simulink model "BMS_Software"  (R2025b)
settings: configuration reference "AutosarConfig" (kept outside this file)
undefined symbols (not defined in the file): BatteryNN, BMS_State_Enum, CntctWaitTime, Contact, currentFactor, CV_Gain, DiscIntNeverNeededParam, HighCellTempLimit, LowCellTempLimit, MaxCellVoltThrsld, MaxChrgCurrLimit, MaxDchrgCurrLimit, MinCellVoltDchrgCurrentLim_BP, MinCellVoltDchrgCurrentLim_Table, noCurrent, OverCellVoltageLimit, PlntBattNumCellPar, PlntBattNumCellSer, PreChrgTimeOut, PreChrgVoltRatio, SOCInit, SRE, ts, UnderCellVoltageLimit, voltThreshold
libraries: simulink x8, BatteryProtection x8, BatteryBalancing x1
settings Model: DataDictionary=BMS_Software_DD.sldd  EnableAccessToBaseWorkspace=off  PauseTimes=0  ExtModeTrigDuration=5  Creator=Chirag Patel  LastModifiedBy=smuckati
settings ConfigSetRef: SourceName=AutosarConfig

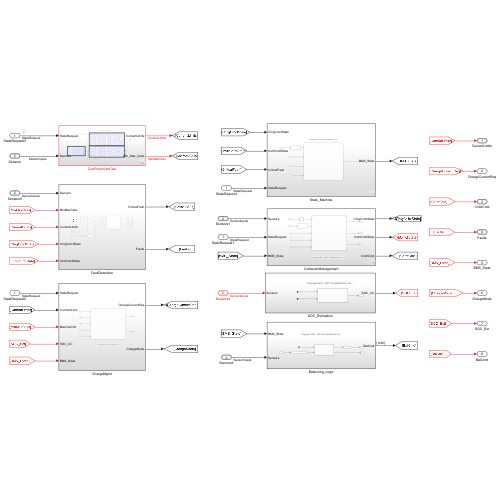
[thumbnail: Simulink's stored preview of the top-level diagram]
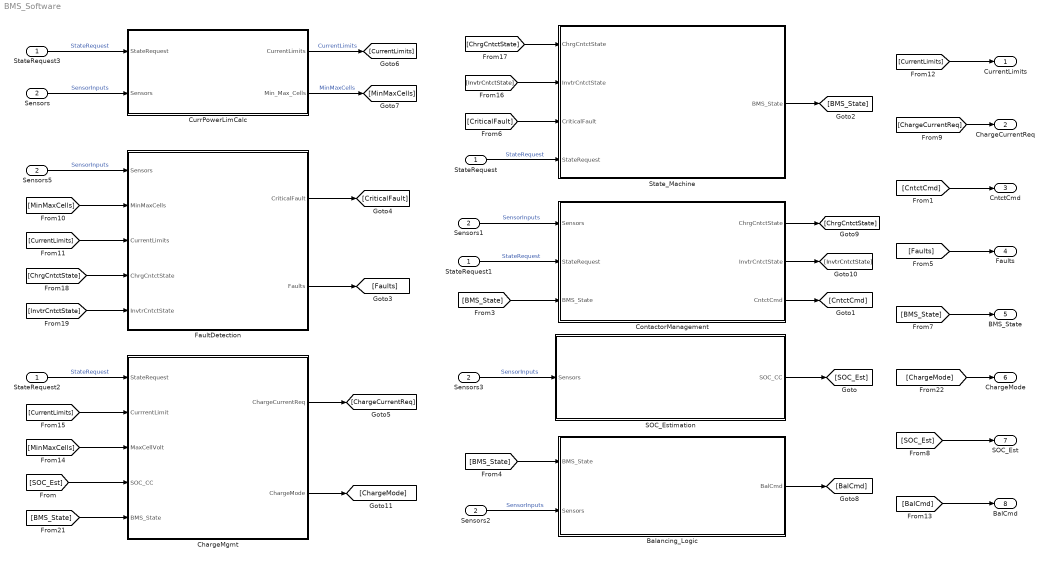
== system BMS_Software ==
  StateRequest : Inport  OutDataTypeStr=Enum: SRE  PortDimensions=1  SampleTime=ts
  Sensors : Inport  Port=2  OutDataTypeStr=Bus: Sensors  BusOutputAsStruct=on
  Balancing_Logic : Subsystem
  ChargeMgmt : Subsystem
  ContactorManagement : Subsystem
  CurrPowerLimCalc : Subsystem
  FaultDetection : Subsystem
  SOC_Estimation : Subsystem
  Sensors{1..3,5} (4 alike) : InportShadow  Port=2  OutDataTypeStr=Bus: Sensors  BusOutputAsStruct=on
  StateRequest1 : InportShadow  OutDataTypeStr=Enum: SRE  PortDimensions=1  SampleTime=ts
  StateRequest2 : InportShadow  OutDataTypeStr=Enum: SRE  PortDimensions=1  SampleTime=ts
  StateRequest3 : InportShadow  OutDataTypeStr=Enum: SRE  PortDimensions=1  SampleTime=ts
  State_Machine : Subsystem
  CurrentLimits : Outport  OutDataTypeStr=Bus: CurrentLimits
  ChargeCurrentReq : Outport  Port=2
  CntctCmd : Outport  Port=3  OutDataTypeStr=Bus: CntctCmd
  Faults : Outport  Port=4  OutDataTypeStr=Bus: Faults
  BMS_State : Outport  Port=5
  ChargeMode : Outport  Port=6
  SOC_Est : Outport  Port=7
  BalCmd : Outport  Port=8
  wires:
  Sensors3/1 -> SOC_Estimation/1(Sensors)  "SensorInputs"
  SOC_Estimation/1(SOC_CC) -> [SOC_Est]
  Sensors2/1 -> Balancing_Logic/2(Sensors)  "SensorInputs"
  [BMS_State] -> Balancing_Logic/1(BMS_State)
  StateRequest1/1 -> ContactorManagement/2(StateRequest)  "StateRequest"
  [BMS_State] -> ContactorManagement/3(BMS_State)
  [CntctCmd] -> CntctCmd/1
  Sensors/1 -> CurrPowerLimCalc/2(Sensors)  "SensorInputs"
  State_Machine/1(BMS_State) -> [BMS_State]
  [Faults] -> Faults/1
  ContactorManagement/3(CntctCmd) -> [CntctCmd]
  StateRequest/1 -> State_Machine/4(StateRequest)  "StateRequest"
  [BMS_State] -> BMS_State/1
  [ChargeCurrentReq] -> ChargeCurrentReq/1
  CurrPowerLimCalc/1(CurrentLimits) -> [CurrentLimits]  "CurrentLimits"
  CurrPowerLimCalc/2(Min_Max_Cells) -> [MinMaxCells]  "MinMaxCells"
  [CurrentLimits] -> CurrentLimits/1
  Balancing_Logic/1(BalCmd) -> [BalCmd]
  ContactorManagement/1(ChrgCntctState) -> [ChrgCntctState]
  ContactorManagement/2(InvtrCntctState) -> [InvtrCntctState]
  [MinMaxCells] -> ChargeMgmt/3(MaxCellVolt)
  [CurrentLimits] -> ChargeMgmt/2(CurrrentLimit)
  StateRequest2/1 -> ChargeMgmt/1(StateRequest)  "StateRequest"
  Sensors1/1 -> ContactorManagement/1(Sensors)  "SensorInputs"
  [SOC_Est] -> ChargeMgmt/4(SOC_CC)
  [ChrgCntctState] -> State_Machine/1(ChrgCntctState)
  [InvtrCntctState] -> State_Machine/2(InvtrCntctState)
  [CriticalFault] -> State_Machine/3(CriticalFault)
  ChargeMgmt/1(ChargeCurrentReq) -> [ChargeCurrentReq]
  ChargeMgmt/2(ChargeMode) -> [ChargeMode]
  [BMS_State] -> ChargeMgmt/5(BMS_State)
  [ChargeMode] -> ChargeMode/1
  [BalCmd] -> BalCmd/1
  [SOC_Est] -> SOC_Est/1
  FaultDetection/1(CriticalFault) -> [CriticalFault]
  FaultDetection/2(Faults) -> [Faults]
  [MinMaxCells] -> FaultDetection/2(MinMaxCells)
  Sensors5/1 -> FaultDetection/1(Sensors)  "SensorInputs"
  [CurrentLimits] -> FaultDetection/3(CurrentLimits)
  [ChrgCntctState] -> FaultDetection/4(ChrgCntctState)
  [InvtrCntctState] -> FaultDetection/5(InvtrCntctState)
  StateRequest3/1 -> CurrPowerLimCalc/1(StateRequest)  "StateRequest"

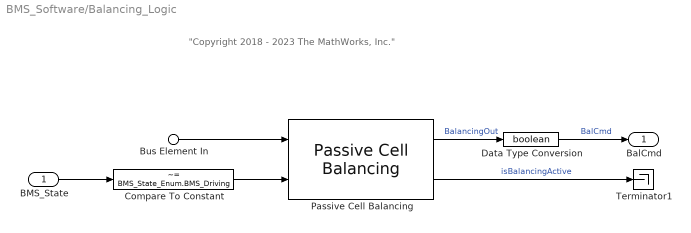
== system BMS_Software/Balancing_Logic ==
  note: "Copyright 2018 - 2023 The MathWorks, Inc."
  BMS_State : Inport  OutDataTypeStr=Enum: BMS_State_Enum  PortDimensions=1  SampleTime=[0.1,0]
  Bus Element In : Inport  Port=2  PortName=Sensors  Element=Cell_Voltages
  Compare To Constant : simulink/Logic and Bit Operations/Compare To Constant  relop=~=  const=BMS_State_Enum.BMS_Driving  OutDataTypeStr=boolean
  Data Type Conversion : DataTypeConversion  OutDataTypeStr=boolean  SaturateOnIntegerOverflow=off  RndMeth=Floor
  Passive Cell Balancing : BatteryBalancing/Passive Cell Balancing  Threshold=0.01  HysteresisBand=0  Td_on=20  Td_off=60  Ts=0.1  dataType=double
      settings: LibrarySourceBlock=batt_sl_lib/Cell Balancing/Passive Cell Balancing
  Terminator1 : Terminator
  BalCmd : Outport  OutDataTypeStr=boolean  PortDimensions=[1,PlntBattNumCellSer]  SampleTime=[0.1,0]  VectorParamsAs1DForOutWhenUnconnected=off
  wires:
  Data Type Conversion/1 -> BalCmd/1  "BalCmd"
  Compare To Constant/1 -> Passive Cell Balancing/2
  Bus Element In/1 -> Passive Cell Balancing/1
  Passive Cell Balancing/1 -> Data Type Conversion/1  "BalancingOut"
  Passive Cell Balancing/2 -> Terminator1/1  "isBalancingActive"
  BMS_State/1 -> Compare To Constant/1

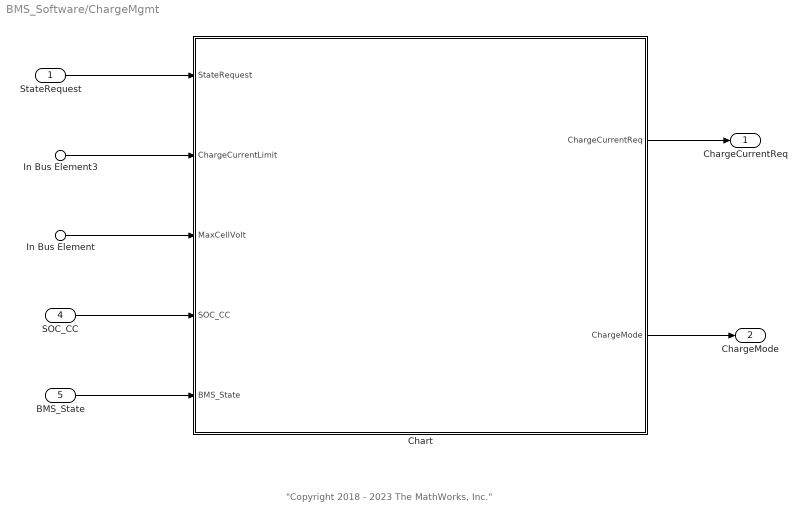
== system BMS_Software/ChargeMgmt ==
  note: "Copyright 2018 - 2023 The MathWorks, Inc."
  StateRequest : Inport  OutDataTypeStr=Enum: SRE  PortDimensions=1
  In Bus Element3 : Inport  Port=2  PortName=CurrrentLimit  Element=ChargeCurrentLimit
  In Bus Element : Inport  Port=3  PortName=MaxCellVolt  Element=MaxCellVolt
  SOC_CC : Inport  Port=4
  BMS_State : Inport  Port=5  OutDataTypeStr=Enum: BMS_State_Enum
  Chart : Stateflow chart  TreatAsAtomicUnit=on
  ChargeCurrentReq : Outport
  ChargeMode : Outport  Port=2
  wires:
  StateRequest/1 -> Chart/1(StateRequest)
  BMS_State/1 -> Chart/5(BMS_State)
  Chart/2(ChargeMode) -> ChargeMode/1
  In Bus Element/1 -> Chart/3(MaxCellVolt)
  Chart/1(ChargeCurrentReq) -> ChargeCurrentReq/1
  In Bus Element3/1 -> Chart/2(ChargeCurrentLimit)
  SOC_CC/1 -> Chart/4(SOC_CC)

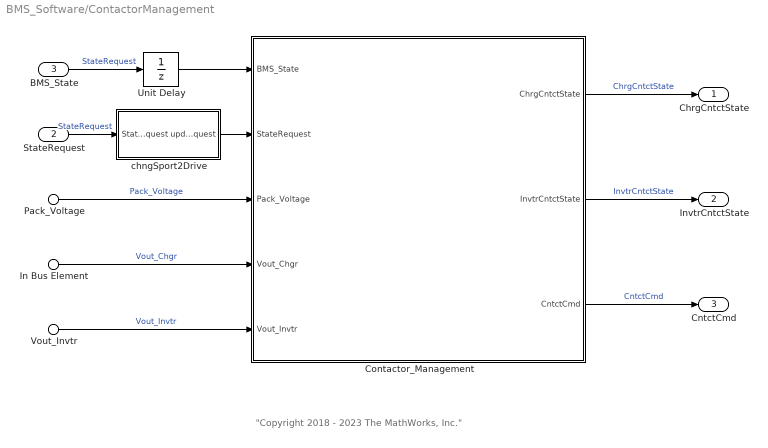
== system BMS_Software/ContactorManagement ==
  note: "Copyright 2018 - 2023 The MathWorks, Inc."
  Pack_Voltage : Inport  PortName=Sensors  Element=Pack_Voltage
  In Bus Element : Inport  PortName=Sensors  Element=Vout_Chgr
  Vout_Invtr : Inport  PortName=Sensors  Element=Vout_Invtr
  StateRequest : Inport  Port=2  OutDataTypeStr=Enum: SRE  PortDimensions=1  SampleTime=[0.10000000000000001,0]
  BMS_State : Inport  Port=3  OutDataTypeStr=Enum: BMS_State_Enum  PortDimensions=1  SampleTime=[0.10000000000000001,0]
  Contactor_Management : Stateflow chart  TreatAsAtomicUnit=on  VariantControl=(default)
  Unit Delay : UnitDelay  InitialCondition=BMS_State_Enum.BMS_Standby  SampleTime=-1  HasFrameUpgradeWarning=on
  chngSport2Drive : Subsystem
  ChrgCntctState : Outport
  InvtrCntctState : Outport  Port=2
  CntctCmd : Outport  Port=3  OutDataTypeStr=Bus: CntctCmd  BusOutputAsStruct=on
  wires:
  Unit Delay/1 -> Contactor_Management/1(BMS_State)
  Pack_Voltage/1 -> Contactor_Management/3(Pack_Voltage)  "Pack_Voltage"
  Vout_Invtr/1 -> Contactor_Management/5(Vout_Invtr)  "Vout_Invtr"
  Contactor_Management/3(CntctCmd) -> CntctCmd/1  "CntctCmd"
  Contactor_Management/1(ChrgCntctState) -> ChrgCntctState/1  "ChrgCntctState"
  In Bus Element/1 -> Contactor_Management/4(Vout_Chgr)  "Vout_Chgr"
  BMS_State/1 -> Unit Delay/1  "StateRequest"
  Contactor_Management/2(InvtrCntctState) -> InvtrCntctState/1  "InvtrCntctState"
  StateRequest/1 -> chngSport2Drive/1(StateRequest)  "StateRequest"
  chngSport2Drive/1(updatedStateRequest) -> Contactor_Management/2(StateRequest)

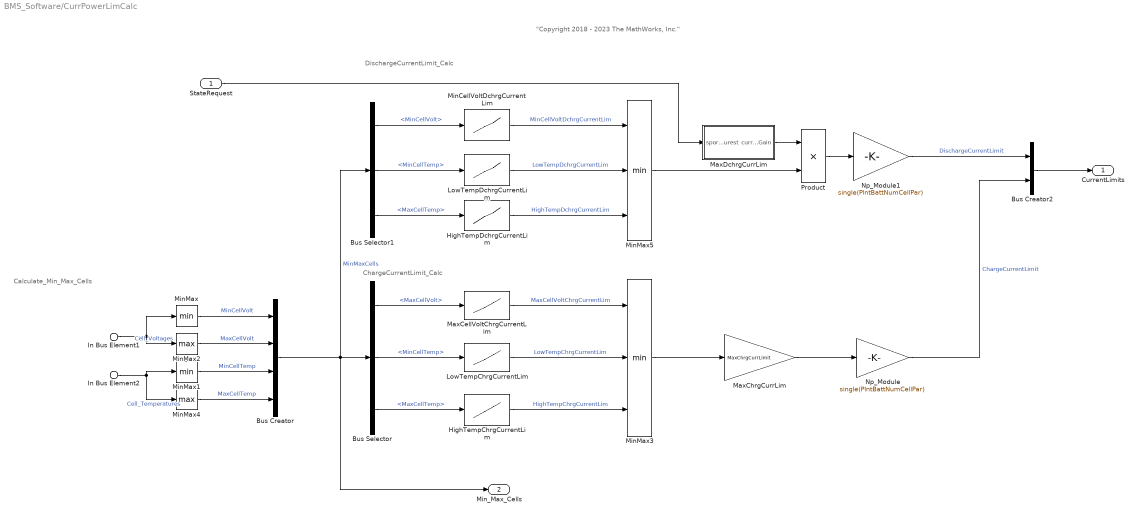
== system BMS_Software/CurrPowerLimCalc ==
  note: ChargeCurrentLimit_Calc
  note: Calculate_Min_Max_Cells
  note: DischargeCurrentLimit_Calc
  note: "Copyright 2018 - 2023 The MathWorks, Inc."
  StateRequest : Inport
  In Bus Element1 : Inport  Port=2  PortName=Sensors  Element=Cell_Voltages
  In Bus Element2 : Inport  Port=2  PortName=Sensors  Element=Cell_Temperatures
  Bus Creator : BusCreator  Inputs=4  OutDataTypeStr=Bus: Min_Max_Cells  NonVirtualBus=on
      settings: InheritFromInputs=off
  Bus Selector : BusSelector  OutputSignals=MaxCellVolt,MinCellTemp,MaxCellTemp
  Bus Selector1 : BusSelector  OutputSignals=MinCellVolt,MinCellTemp,MaxCellTemp
  Bus Creator2 : BusCreator  Inputs=2  OutDataTypeStr=Bus: CurrentLimits  NonVirtualBus=on
  HighTempChrgCurrentLim : Lookup_n-D  NumberOfTableDimensions=1  BreakpointsForDimension1="single([40  45  50    55 65])"  Table=single([1.0 1.0 0.75 0.5 0])  ExtrapMethod=Clip  InternalRulePriority=Speed  RndMeth=Simplest
  HighTempDchrgCurrentLim : Lookup_n-D  NumberOfTableDimensions=1  BreakpointsForDimension1=single([40, 45, 50, 60])  Table=single([1, 0.5, 0.3, 0])  ExtrapMethod=Clip  InternalRulePriority=Speed  RndMeth=Simplest
  LowTempChrgCurrentLim : Lookup_n-D  NumberOfTableDimensions=1  BreakpointsForDimension1=single([-15 -10 -5.0 0.0 5.0 10 15.0])  Table="single([0.1 0.2  0.3 0.3 0.5 1.0 1.0])"  ExtrapMethod=Clip  InternalRulePriority=Speed  RndMeth=Simplest
  LowTempDchrgCurrentLim : Lookup_n-D  NumberOfTableDimensions=1  BreakpointsForDimension1="single([-10, -5,    0,   5, 10, 15, 20])"  Table="single([0,  0.2, 0.3, 0.5, 0.75, 1, 1])"  ExtrapMethod=Clip  InternalRulePriority=Speed  RndMeth=Simplest
  MaxCellVoltChrgCurrentLim : Lookup_n-D  NumberOfTableDimensions=1  BreakpointsForDimension1=single([4.0 4.10 4.15 4.2])  Table=single([1.0 0.75 0.50 0.2])  ExtrapMethod=Clip  InternalRulePriority=Speed  RndMeth=Simplest
  MaxChrgCurrLim : Gain  Gain=MaxChrgCurrLimit
  MaxDchrgCurrLim : Subsystem
  MinCellVoltDchrgCurrentLim : Lookup_n-D  NumberOfTableDimensions=1  DataSpecification=Lookup table object  LookupTableObject=MinCellVoltDchrgCurrentLimTable  BreakpointsForDimension1=MinCellVoltDchrgCurrentLim_BP  Table=MinCellVoltDchrgCurrentLim_Table  ExtrapMethod=Clip  InternalRulePriority=Speed  RndMeth=Simplest
  MinMax : MinMax
  MinMax1 : MinMax
  MinMax2 : MinMax  Function=max
  MinMax3 : MinMax  Inputs=3
  MinMax4 : MinMax  Function=max
  MinMax5 : MinMax  Inputs=3
  Np_Module : Gain  Gain=single(PlntBattNumCellPar)  ParamDataTypeStr=Inherit: Inherit from 'Gain'
  Np_Module1 : Gain  Gain=single(PlntBattNumCellPar)  ParamDataTypeStr=Inherit: Inherit from 'Gain'
  Product : Product
  CurrentLimits : Outport  OutDataTypeStr=Bus: CurrentLimits
  Min_Max_Cells : Outport  Port=2  OutDataTypeStr=Bus: Min_Max_Cells
  wires:
  Bus Selector/2 -> LowTempChrgCurrentLim/1  "<MinCellTemp>"
  In Bus Element2/1 -> MinMax4/1, MinMax1/1  "Cell_Temperatures"
  MinMax/1 -> Bus Creator/1  "MinCellVolt"
  Np_Module1/1 -> Bus Creator2/1  "DischargeCurrentLimit"
  MinMax4/1 -> Bus Creator/4  "MaxCellTemp"
  MinMax2/1 -> Bus Creator/2  "MaxCellVolt"
  Bus Creator/1 -> Min_Max_Cells/1, Bus Selector1/1, Bus Selector/1  "MinMaxCells"
  MaxChrgCurrLim/1 -> Np_Module/1
  LowTempDchrgCurrentLim/1 -> MinMax5/2  "LowTempDchrgCurrentLim"
  HighTempDchrgCurrentLim/1 -> MinMax5/3  "HighTempDchrgCurrentLim"
  Bus Selector1/2 -> LowTempDchrgCurrentLim/1  "<MinCellTemp>"
  In Bus Element1/1 -> MinMax/1, MinMax2/1  "Cell_Voltages"
  HighTempChrgCurrentLim/1 -> MinMax3/3  "HighTempChrgCurrentLim"
  MinMax3/1 -> MaxChrgCurrLim/1
  Bus Selector1/1 -> MinCellVoltDchrgCurrentLim/1  "<MinCellVolt>"
  MaxCellVoltChrgCurrentLim/1 -> MinMax3/1  "MaxCellVoltChrgCurrentLim"
  LowTempChrgCurrentLim/1 -> MinMax3/2  "LowTempChrgCurrentLim"
  MinMax1/1 -> Bus Creator/3  "MinCellTemp"
  Bus Selector/1 -> MaxCellVoltChrgCurrentLim/1  "<MaxCellVolt>"
  Bus Selector/3 -> HighTempChrgCurrentLim/1  "<MaxCellTemp>"
  Bus Creator2/1 -> CurrentLimits/1
  MinMax5/1 -> Product/2
  Product/1 -> Np_Module1/1
  MinCellVoltDchrgCurrentLim/1 -> MinMax5/1  "MinCellVoltDchrgCurrentLim"
  Np_Module/1 -> Bus Creator2/2  "ChargeCurrentLimit"
  Bus Selector1/3 -> HighTempDchrgCurrentLim/1  "<MaxCellTemp>"
  StateRequest/1 -> MaxDchrgCurrLim/1(sportMode_requrest)
  MaxDchrgCurrLim/1(currentDchargGain) -> Product/1

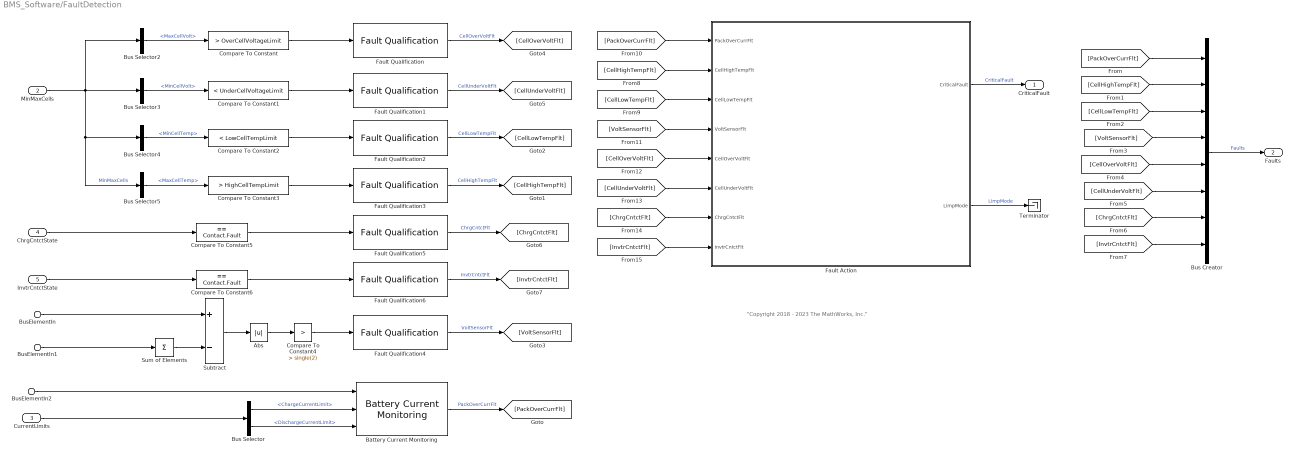
== system BMS_Software/FaultDetection ==
  note: "Copyright 2018 - 2023 The MathWorks, Inc."
  BusElementIn1 : Inport  PortName=Sensors  Element=Cell_Voltages
  BusElementIn : Inport  PortName=Sensors  Element=Pack_Voltage
  BusElementIn2 : Inport  PortName=Sensors  Element=Pack_Current
  MinMaxCells : Inport  Port=2  OutDataTypeStr=Bus: Min_Max_Cells
  CurrentLimits : Inport  Port=3  OutDataTypeStr=Bus: CurrentLimits
  ChrgCntctState : Inport  Port=4  OutDataTypeStr=Enum: Contact
  InvtrCntctState : Inport  Port=5  OutDataTypeStr=Enum: Contact
  Abs : Abs  SaturateOnIntegerOverflow=off
  Battery Current Monitoring : BatteryProtection/Battery Current Monitoring  ErrorLimit=0  QualTime=2  DisqualTime=4  Ts=0.1  DataType=Inherit: auto
      settings: LibrarySourceBlock=|
      | batt_sl_lib/Protection/Battery Current
      | Monitoring
  Bus Creator : BusCreator  Inputs=8  OutDataTypeStr=Bus: Faults  NonVirtualBus=on
      settings: InheritFromInputs=off
  Bus Selector : BusSelector  OutputSignals=ChargeCurrentLimit,DischargeCurrentLimit
  Bus Selector2 : BusSelector  OutputSignals=MaxCellVolt
  Bus Selector3 : BusSelector  OutputSignals=MinCellVolt
  Bus Selector4 : BusSelector  OutputSignals=MinCellTemp
  Bus Selector5 : BusSelector  OutputSignals=MaxCellTemp
  Compare To Constant : simulink/Logic and Bit Operations/Compare To Constant  relop=>  const=OverCellVoltageLimit  OutDataTypeStr=boolean
  Compare To Constant1 : simulink/Logic and Bit Operations/Compare To Constant  relop=<  const=UnderCellVoltageLimit  OutDataTypeStr=boolean
  Compare To Constant2 : simulink/Logic and Bit Operations/Compare To Constant  relop=<  const=LowCellTempLimit  OutDataTypeStr=boolean
  Compare To Constant3 : simulink/Logic and Bit Operations/Compare To Constant  relop=>  const=HighCellTempLimit  OutDataTypeStr=boolean
  Compare To Constant4 : simulink/Logic and Bit Operations/Compare To Constant  relop=>  const=single(2)  OutDataTypeStr=boolean
  Compare To Constant5 : simulink/Logic and Bit Operations/Compare To Constant  relop===  const=Contact.Fault  OutDataTypeStr=boolean
  Compare To Constant6 : simulink/Logic and Bit Operations/Compare To Constant  relop===  const=Contact.Fault  OutDataTypeStr=boolean
  Fault Action : Truth Table  TreatAsAtomicUnit=on
  Fault Qualification : BatteryProtection/Fault Qualification  QualTime=2  DisqualTime=4  Ts=0.1
      settings: LibrarySourceBlock=batt_sl_lib/Protection/Fault Qualification
  Fault Qualification1 : BatteryProtection/Fault Qualification  QualTime=2  DisqualTime=4  Ts=0.1
      settings: LibrarySourceBlock=batt_sl_lib/Protection/Fault Qualification
  Fault Qualification2 : BatteryProtection/Fault Qualification  QualTime=4  DisqualTime=6  Ts=0.1
      settings: LibrarySourceBlock=batt_sl_lib/Protection/Fault Qualification
  Fault Qualification3 : BatteryProtection/Fault Qualification  QualTime=4  DisqualTime=6  Ts=0.1
      settings: LibrarySourceBlock=batt_sl_lib/Protection/Fault Qualification
  Fault Qualification4 : BatteryProtection/Fault Qualification  QualTime=2  DisqualTime=4  Ts=0.1
      settings: LibrarySourceBlock=batt_sl_lib/Protection/Fault Qualification
  Fault Qualification5 : BatteryProtection/Fault Qualification  QualTime=0.5  DisqualTime=2  Ts=0.1
      settings: LibrarySourceBlock=batt_sl_lib/Protection/Fault Qualification
  Fault Qualification6 : BatteryProtection/Fault Qualification  QualTime=0.5  DisqualTime=2  Ts=0.1
      settings: LibrarySourceBlock=batt_sl_lib/Protection/Fault Qualification
  Subtract : Sum  Inputs=+-
  Sum of Elements : Sum  Inputs=+
  Terminator : Terminator
  CriticalFault : Outport
  Faults : Outport  Port=2  OutDataTypeStr=Bus: Faults
  wires:
  [InvtrCntctFlt] -> Fault Action/8(InvtrCntctFlt)
  Bus Selector4/1 -> Compare To Constant2/1  "<MinCellTemp>"
  Abs/1 -> Compare To Constant4/1
  BusElementIn2/1 -> Battery Current Monitoring/1
  [CellHighTempFlt] -> Fault Action/2(CellHighTempFlt)
  Fault Qualification1/1 -> [CellUnderVoltFlt]  "CellUnderVoltFlt"
  [CellUnderVoltFlt] -> Bus Creator/6
  Fault Qualification4/1 -> [VoltSensorFlt]  "VoltSensorFlt"
  Compare To Constant2/1 -> Fault Qualification2/1
  Compare To Constant1/1 -> Fault Qualification1/1
  Bus Selector2/1 -> Compare To Constant/1  "<MaxCellVolt>"
  Bus Selector5/1 -> Compare To Constant3/1  "<MaxCellTemp>"
  Fault Qualification5/1 -> [ChrgCntctFlt]  "ChrgCntctFlt"
  [ChrgCntctFlt] -> Bus Creator/7
  Compare To Constant6/1 -> Fault Qualification6/1
  [CellLowTempFlt] -> Bus Creator/3
  Fault Action/2(LimpMode) -> Terminator/1  "LimpMode"
  ChrgCntctState/1 -> Compare To Constant5/1
  CurrentLimits/1 -> Bus Selector/1
  InvtrCntctState/1 -> Compare To Constant6/1
  [VoltSensorFlt] -> Bus Creator/4
  [CellHighTempFlt] -> Bus Creator/2
  Fault Qualification6/1 -> [InvtrCntctFlt]  "InvtrCntctFlt"
  MinMaxCells/1 -> Bus Selector5/1, Bus Selector4/1, Bus Selector3/1, Bus Selector2/1  "MinMaxCells"
  [PackOverCurrFlt] -> Fault Action/1(PackOverCurrFlt)
  [PackOverCurrFlt] -> Bus Creator/1
  [CellOverVoltFlt] -> Fault Action/5(CellOverVoltFlt)
  [VoltSensorFlt] -> Fault Action/4(VoltSensorFlt)
  Compare To Constant3/1 -> Fault Qualification3/1
  [CellLowTempFlt] -> Fault Action/3(CellLowTempFlt)
  [InvtrCntctFlt] -> Bus Creator/8
  Bus Selector/1 -> Battery Current Monitoring/2  "<ChargeCurrentLimit>"
  Fault Qualification3/1 -> [CellHighTempFlt]  "CellHighTempFlt"
  [CellOverVoltFlt] -> Bus Creator/5
  Compare To Constant4/1 -> Fault Qualification4/1
  BusElementIn/1 -> Subtract/1
  Fault Action/1(CriticalFault) -> CriticalFault/1  "CriticalFault"
  Bus Selector3/1 -> Compare To Constant1/1  "<MinCellVolt>"
  Battery Current Monitoring/1 -> [PackOverCurrFlt]  "PackOverCurrFlt"
  Bus Creator/1 -> Faults/1  "Faults"
  Bus Selector/2 -> Battery Current Monitoring/3  "<DischargeCurrentLimit>"
  [ChrgCntctFlt] -> Fault Action/7(ChrgCntctFlt)
  Compare To Constant/1 -> Fault Qualification/1
  Subtract/1 -> Abs/1
  [CellUnderVoltFlt] -> Fault Action/6(CellUnderVoltFlt)
  Sum of Elements/1 -> Subtract/2
  BusElementIn1/1 -> Sum of Elements/1
  Fault Qualification/1 -> [CellOverVoltFlt]  "CellOverVoltFlt"
  Compare To Constant5/1 -> Fault Qualification5/1
  Fault Qualification2/1 -> [CellLowTempFlt]  "CellLowTempFlt"

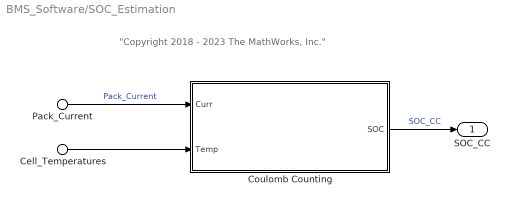
== system BMS_Software/SOC_Estimation ==
  note: "Copyright 2018 - 2023 The MathWorks, Inc."
  Pack_Current : Inport  PortName=Sensors  Element=Pack_Current
  Cell_Temperatures : Inport  PortName=Sensors  Element=Cell_Temperatures
  Coulomb Counting : Subsystem  VariantControl=SocAlgo==1
  SOC_CC : Outport
  wires:
  Cell_Temperatures/1 -> Coulomb Counting/2(Temp)
  Pack_Current/1 -> Coulomb Counting/1(Curr)  "Pack_Current"
  Coulomb Counting/1(SOC) -> SOC_CC/1  "SOC_CC"

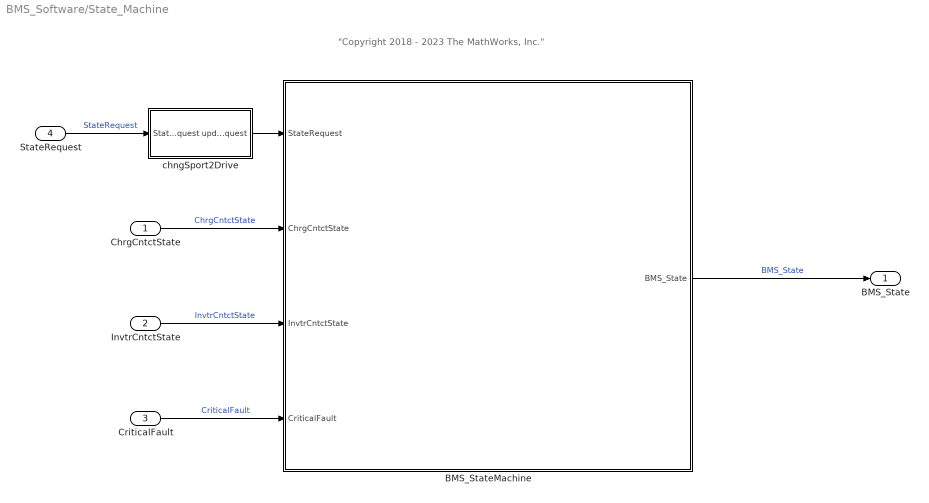
== system BMS_Software/State_Machine ==
  note: "Copyright 2018 - 2023 The MathWorks, Inc."
  ChrgCntctState : Inport
  InvtrCntctState : Inport  Port=2
  CriticalFault : Inport  Port=3
  StateRequest : Inport  Port=4  OutDataTypeStr=Enum: SRE  PortDimensions=1  SampleTime=[0.10000000000000001,0]  Interpolate=off
  BMS_StateMachine : Stateflow chart  TreatAsAtomicUnit=on  VariantControl=(default)
  chngSport2Drive : Subsystem
  BMS_State : Outport  OutDataTypeStr=Enum: BMS_State_Enum  PortDimensions=1  SampleTime=[0.10000000000000001,0]  VectorParamsAs1DForOutWhenUnconnected=off
  wires:
  InvtrCntctState/1 -> BMS_StateMachine/3(InvtrCntctState)  "InvtrCntctState"
  ChrgCntctState/1 -> BMS_StateMachine/2(ChrgCntctState)  "ChrgCntctState"
  CriticalFault/1 -> BMS_StateMachine/4(CriticalFault)  "CriticalFault"
  StateRequest/1 -> chngSport2Drive/1(StateRequest)  "StateRequest"
  BMS_StateMachine/1(BMS_State) -> BMS_State/1  "BMS_State"
  chngSport2Drive/1(updatedStateRequest) -> BMS_StateMachine/1(StateRequest)

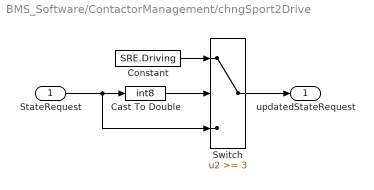
== system BMS_Software/ContactorManagement/chngSport2Drive ==
  StateRequest : Inport
  Cast To Double : DataTypeConversion  OutDataTypeStr=int8  SaturateOnIntegerOverflow=off  RndMeth=Floor
  Constant : Constant  Value=SRE.Driving
  Switch : Switch  Threshold=3  SaturateOnIntegerOverflow=off  InputSameDT=off
  updatedStateRequest : Outport
  wires:
  Switch/1 -> updatedStateRequest/1
  Cast To Double/1 -> Switch/2
  StateRequest/1 -> Switch/3, Cast To Double/1
  Constant/1 -> Switch/1

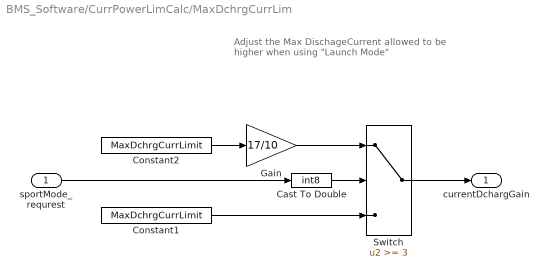
== system BMS_Software/CurrPowerLimCalc/MaxDchrgCurrLim ==
  note: Adjust the Max DischageCurrent allowed to be higher when using "Launch Mode"
  sportMode_requrest : Inport
  Cast To Double : DataTypeConversion  OutDataTypeStr=int8  SaturateOnIntegerOverflow=off  RndMeth=Floor
  Constant1 : Constant  Value=MaxDchrgCurrLimit
  Constant2 : Constant  Value=MaxDchrgCurrLimit
  Gain : Gain  Gain=17/10
  Switch : Switch  Threshold=3  SaturateOnIntegerOverflow=off  InputSameDT=off
  currentDchargGain : Outport
  wires:
  Constant1/1 -> Switch/3
  Gain/1 -> Switch/1
  sportMode_requrest/1 -> Cast To Double/1
  Cast To Double/1 -> Switch/2
  Switch/1 -> currentDchargGain/1
  Constant2/1 -> Gain/1

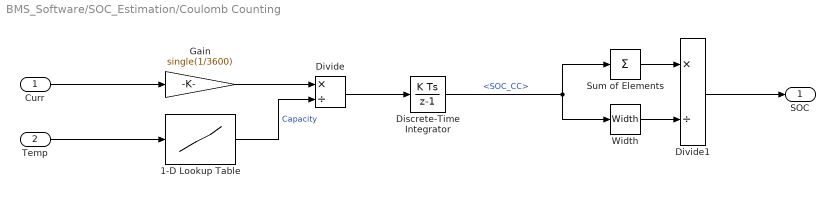
== system BMS_Software/SOC_Estimation/Coulomb Counting ==
  Curr : Inport
  Temp : Inport  Port=2
  1-D Lookup Table : Lookup_n-D  NumberOfTableDimensions=1  BreakpointsForDimension1=single(BatteryNN(1).T_vec)  Table=single(BatteryNN(1).AH)*PlntBattNumCellPar  InternalRulePriority=Speed  RndMeth=Simplest
  Discrete-Time Integrator : DiscreteIntegrator  InitialCondition=ones(1,PlntBattNumCellSer)*single(SOCInit)  SampleTime=-1  LimitOutput=on  UpperSaturationLimit=1  LowerSaturationLimit=0  ICPrevOutput=DiscIntNeverNeededParam  ICPrevScaledInput=DiscIntNeverNeededParam
  Divide : Product  Inputs=*/
  Divide1 : Product  Inputs=*/
  Gain : Gain  Gain=single(1/3600)
  Sum of Elements : Sum  Inputs=+
  Width : Width  DataType=single
  SOC : Outport  VectorParamsAs1DForOutWhenUnconnected=off
  wires:
  Curr/1 -> Gain/1
  Gain/1 -> Divide/1
  Divide/1 -> Discrete-Time Integrator/1
  1-D Lookup Table/1 -> Divide/2  "Capacity"
  Temp/1 -> 1-D Lookup Table/1
  Sum of Elements/1 -> Divide1/1
  Width/1 -> Divide1/2
  Divide1/1 -> SOC/1
  Discrete-Time Integrator/1 -> Width/1, Sum of Elements/1  "<SOC_CC>"

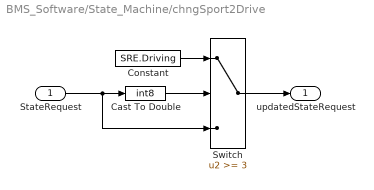
== system BMS_Software/State_Machine/chngSport2Drive ==
  StateRequest : Inport
  Cast To Double : DataTypeConversion  OutDataTypeStr=int8  SaturateOnIntegerOverflow=off  RndMeth=Floor
  Constant : Constant  Value=SRE.Driving
  Switch : Switch  Threshold=3  SaturateOnIntegerOverflow=off  InputSameDT=off
  updatedStateRequest : Outport
  wires:
  Switch/1 -> updatedStateRequest/1
  Cast To Double/1 -> Switch/2
  StateRequest/1 -> Switch/3, Cast To Double/1
  Constant/1 -> Switch/1

== stateflow chart BMS_Software/State_Machine/BMS_StateMachine ==
  state Driving
    en:
    BMS_State = ...
    BMS_State_Enum.BMS_Driving;
  state Standby
    en:
    BMS_State = ...
    BMS_State_Enum.BMS_Standby;
  state Charging
    en:
    BMS_State = ...
    BMS_State_Enum.BMS_Charging;
  state Fault
    en,du:
    BMS_State = BMS_State_Enum.BMS_Fault;
  (default) -> Standby
  Standby -> Charging [order 1] : [StateRequest ==SRE.Charging...
      | && ChrgCntctState == Contact.Close]
  Standby -> Driving [order 3] : [StateRequest == SRE.Driving && ...
      | InvtrCntctState == Contact.Close]
  Charging -> Standby [order 2] : [StateRequest ~=SRE.Charging...
      | || ChrgCntctState ~= Contact.Close]
  Driving -> Standby [order 2] : [StateRequest ~= SRE.Driving || ...
      | InvtrCntctState ~= Contact.Close]
  Driving -> Fault [order 1] : [CriticalFault]
  Standby -> Fault [order 2] : [CriticalFault]
  Fault -> Standby : [~CriticalFault]
  Charging -> Fault [order 1] : [CriticalFault]
  data: StateRequest input Enum: SRE; BMS_State output Enum: BMS_State_Enum =BMS_State_Enum.BMS_Standby; ChrgCntctState input Enum: Contact; InvtrCntctState input Enum: Contact; CriticalFault input boolean

== matlab function BMS_Software/FaultDetection/Fault Action ==
  data: PackOverCurrFlt input; CriticalFault output boolean size=1 =false; CellHighTempFlt input; CellLowTempFlt input; VoltSensorFlt input; CellOverVoltFlt input; CellUnderVoltFlt input; ChrgCntctFlt input; InvtrCntctFlt input; LimpMode output boolean =false
function [CriticalFault, LimpMode] = fcn(PackOverCurrFlt, CellHighTempFlt, CellLowTempFlt, VoltSensorFlt, CellOverVoltFlt, CellUnderVoltFlt, ChrgCntctFlt, InvtrCntctFlt)

aVarTruthTableCondition_1 = false;
aVarTruthTableCondition_2 = false;


% Any Non-Critical Fault Active

aVarTruthTableCondition_1 = logical(PackOverCurrFlt || CellHighTempFlt || CellLowTempFlt || CellOverVoltFlt || CellUnderVoltFlt ||   VoltSensorFlt);

% Critical Fault Active

aVarTruthTableCondition_2 = logical(ChrgCntctFlt || InvtrCntctFlt);

if (aVarTruthTableCondition_1)
    aFcnTruthTableAction_3();
elseif (aVarTruthTableCondition_2)
    aFcnTruthTableAction_2();
else % Default
    aFcnTruthTableAction_1();
end

function aFcnTruthTableAction_1()

% No Fault Not Present

CriticalFault = false;
LimpMode = false;

function aFcnTruthTableAction_2()

% Critical Fault Present

CriticalFault = true;

function aFcnTruthTableAction_3()

% Limp Mode Active

LimpMode = true;

== stateflow chart BMS_Software/ContactorManagement/Contactor_Management ==
  state ChrgCntctSt [parallel]
    settings: executionOrder=1
    state CloseChgrCntct
      state CloseNegCntct
        CntctCmd.NegCntctChgrCmd = true;
      state PreChrgFlt
        ChrgCntctState = Contact.Fault;
      state ClosePreChrgRly
        CntctCmd.PreChrgRelayChgrCmd = true;
      state ClosePosCntct
        CntctCmd.PosCntctChgrCmd = true;
      state OpenPreChrgRly
        CntctCmd.PreChrgRelayChgrCmd = false;
        ChrgCntctState = Contact.Close;
      (default) -> ChrgCntctSt.CloseChgrCntct.CloseNegCntct : {ChrgCntctState = Contact.Init;}
      ChrgCntctSt.CloseChgrCntct.CloseNegCntct -> ChrgCntctSt.CloseChgrCntct.ClosePreChrgRly : after(CntctWaitTime,msec)
      ChrgCntctSt.CloseChgrCntct.ClosePreChrgRly -> ChrgCntctSt.CloseChgrCntct.PreChrgFlt [order 1] : after(PreChrgTimeOut,sec)
          | % Check timeout
      ChrgCntctSt.CloseChgrCntct.ClosePreChrgRly -> ChrgCntctSt.CloseChgrCntct.ClosePosCntct [order 2] : [Vout_Chgr/Pack_Voltage >=PreChrgVoltRatio]
      ChrgCntctSt.CloseChgrCntct.ClosePosCntct -> ChrgCntctSt.CloseChgrCntct.OpenPreChrgRly : after(CntctWaitTime,msec)
    state OpenChgrCntct
      state ClosePreChrgRly
        CntctCmd.PreChrgRelayChgrCmd = true;
      state OpenPosCntct
        CntctCmd.PosCntctChgrCmd = false;
      state OpenPreChrgRly
        CntctCmd.PreChrgRelayChgrCmd = false;
      state OpenNegCntct
        CntctCmd.NegCntctChgrCmd = false;
        ChrgCntctState = Contact.Open;
      (default) -> ChrgCntctSt.OpenChgrCntct.ClosePreChrgRly : {ChrgCntctState = Contact.Init;}
      ChrgCntctSt.OpenChgrCntct.ClosePreChrgRly -> ChrgCntctSt.OpenChgrCntct.OpenPosCntct : after(CntctWaitTime,msec)
          | % Check for low current
      ChrgCntctSt.OpenChgrCntct.OpenPosCntct -> ChrgCntctSt.OpenChgrCntct.OpenPreChrgRly : after(CntctWaitTime,msec)
      ChrgCntctSt.OpenChgrCntct.OpenPreChrgRly -> ChrgCntctSt.OpenChgrCntct.OpenNegCntct : after(CntctWaitTime,msec)
    (default) -> OpenChgrCntct : {ChrgCntctState = Contact.Init;}
    CloseChgrCntct -> OpenChgrCntct : [StateRequest ~= SRE.Charging || ...
        | BMS_State == BMS_State_Enum.BMS_Fault]
    OpenChgrCntct -> CloseChgrCntct : [StateRequest == SRE.Charging && ...
        | InvtrCntctState == Contact.Open && ...
        | BMS_State ~= BMS_State_Enum.BMS_Fault]
  state InvtrCntctSt [parallel]
    settings: executionOrder=2
    state OpenInvtrCntct
      state ClosePreChrgRly
        CntctCmd.PreChrgRelayInvtrCmd = true;
      state OpenPosCntct
        CntctCmd.PosCntctInvtrCmd = false;
      state OpenPreChrgRly
        CntctCmd.PreChrgRelayInvtrCmd = false;
      state OpenNegCntct
        CntctCmd.NegCntctInvtrCmd = false;
        InvtrCntctState = Contact.Open;
      (default) -> InvtrCntctSt.OpenInvtrCntct.ClosePreChrgRly : {InvtrCntctState = Contact.Init;}
      InvtrCntctSt.OpenInvtrCntct.ClosePreChrgRly -> InvtrCntctSt.OpenInvtrCntct.OpenPosCntct : after(CntctWaitTime,msec)
          | % Check for low current
      InvtrCntctSt.OpenInvtrCntct.OpenPosCntct -> InvtrCntctSt.OpenInvtrCntct.OpenPreChrgRly : after(CntctWaitTime,msec)
      InvtrCntctSt.OpenInvtrCntct.OpenPreChrgRly -> InvtrCntctSt.OpenInvtrCntct.OpenNegCntct : after(CntctWaitTime,msec)
    state CloseInvtrCntct
      state CloseNegCntct
        CntctCmd.NegCntctInvtrCmd = true;
      state ClosePreChrgRly
        CntctCmd.PreChrgRelayInvtrCmd = true;
      state PreChrgFlt
        InvtrCntctState = Contact.Fault;
      state ClosePosCntct
        CntctCmd.PosCntctInvtrCmd = true;
      state OpenPreChrgRly
        CntctCmd.PreChrgRelayInvtrCmd = false;
        InvtrCntctState = Contact.Close;
      (default) -> InvtrCntctSt.CloseInvtrCntct.CloseNegCntct : {InvtrCntctState = Contact.Init;}
      InvtrCntctSt.CloseInvtrCntct.CloseNegCntct -> InvtrCntctSt.CloseInvtrCntct.ClosePreChrgRly : after(CntctWaitTime,msec)
      InvtrCntctSt.CloseInvtrCntct.ClosePreChrgRly -> InvtrCntctSt.CloseInvtrCntct.PreChrgFlt [order 1] : after(PreChrgTimeOut,sec)
          | % Check timeout
      InvtrCntctSt.CloseInvtrCntct.ClosePreChrgRly -> InvtrCntctSt.CloseInvtrCntct.ClosePosCntct [order 2] : [Vout_Invtr/Pack_Voltage >=PreChrgVoltRatio]
      InvtrCntctSt.CloseInvtrCntct.ClosePosCntct -> InvtrCntctSt.CloseInvtrCntct.OpenPreChrgRly : after(CntctWaitTime,msec)
    (default) -> OpenInvtrCntct : {InvtrCntctState =Contact.Init;}
    CloseInvtrCntct -> OpenInvtrCntct : [StateRequest ~= SRE.Driving || ...
        | BMS_State == BMS_State_Enum.BMS_Fault]
    OpenInvtrCntct -> CloseInvtrCntct : [StateRequest == SRE.Driving && ...
        | ChrgCntctState == Contact.Open && ...
        | BMS_State ~= BMS_State_Enum.BMS_Fault]
  data: BMS_State input; StateRequest input Enum: SRE; Pack_Voltage input single; Vout_Chgr input single; Vout_Invtr input single; CntctWaitTime parameter uint16; PreChrgTimeOut parameter uint8; PreChrgVoltRatio parameter single; ChrgCntctState output Enum: Contact; InvtrCntctState output Enum: Contact; CntctCmd output Bus: CntctCmd

== stateflow chart BMS_Software/ChargeMgmt/Chart ==
  state ChrgStandby
    en:
    ChargeMode = ChargeMode_Enum.ChrgStandby;
    ChargeCurrentReq = noCurrent;
  state ChrgCC
    en:
    ChargeMode = ChargeMode_Enum.CC;
    du:
    ChargeCurrentReq = ChargeCurrentLimit;
  state ChrgCV
    en:
    ChargeMode = ChargeMode_Enum.CV;
    du:
    ChargeCurrentReq = ChargeCurrentReq - CV_Gain*(MaxCellVolt - MaxCellVoltThrsld);
    ChargeCurrentReq = min(ChargeCurrentReq, ChargeCurrentLimit);
  (default) -> ChrgStandby
  ChrgCV -> ChrgStandby : [StateRequest ~= SRE.Charging || ...
      | ChargeCurrentReq <= (MaxChrgCurrLimit*PlntBattNumCellPar/currentFactor) || ...
      | max(SOC_CC) >single(0.98)]
  ChrgCC -> ChrgStandby [order 1] : [StateRequest ~= SRE.Charging]
  ChrgStandby -> ChrgCC : [StateRequest == SRE.Charging && ...
      | BMS_State == BMS_State_Enum.BMS_Charging && ...
      | MaxCellVolt < voltThreshold && ...
      | max(SOC_CC) < single(0.95)]
  ChrgCC -> ChrgCV [order 2] : [MaxCellVolt>=...
      | MaxCellVoltThrsld]
  data: StateRequest input; ChargeCurrentLimit input; MaxCellVolt input; SOC_CC input; ChargeCurrentReq output; CV_Gain parameter; voltThreshold parameter; noCurrent parameter; MaxCellVoltThrsld parameter; PlntBattNumCellPar parameter; currentFactor parameter; MaxChrgCurrLimit parameter; ChargeMode output; BMS_State input
